simulink model "stellaris_lp_overrun"  (R2017a)
settings: Solver=ode3  StartTime=0.0  StopTime=10.0  FixedStep=1/30e3  RelTol=1e-3
libraries: stellaris_lp_lib x3, simulink x3
settings Model: ExtModeTrigDuration=2  Creator=peselnikmg  LastModifiedBy=Nilim
settings DataIOCC: LimitDataPoints=on  SaveFormat=Array  SignalLoggingSaveFormat=ModelDataLogs
settings OptimizationCC: PassReuseOutputArgsAs=Individual arguments  ExpressionDepthLimit=2147483647  MaxStackSize=64
settings DebuggingCC: ParameterTunabilityLossMsg=error  StateNameClashWarn=warning  SFUnexpectedBacktrackingDiag=warning  SFNoUnconditionalDefaultTransitionDiag=warning  SFExecutionAtInitializationDiag=none
settings HardwareCC: ProdBitPerPointer=32  ProdBitPerSizeT=32  ProdBitPerPtrDiffT=32  ProdLargestAtomicInteger=Long  ProdLargestAtomicFloat=Double  ProdWordSize=32  ProdHWDeviceType=ARM Compatible->ARM Cortex
settings ModelReferenceCC: PropagateSignalLabelsOutOfModel=off
settings SFSimCC: MATLABDynamicMemAlloc=off
settings RTWCC: SystemTargetFile=ert.tlc  HardwareBoard=Tiva TM4C123G Launchpad  TLCOptions=-aInlineSetEventsForThisBaseRateFcn=TLC_FALSE -aSuppressMultiTaskScheduler=TLC_FALSE -aRateBasedStepFcn=1  TemplateMakefile=ert_default_tmf  Description=Embedded Coder  GenerateReport=on  RTWVerbose=off  Toolchain=Texas Instruments Code Composer Studio (Tiva)  IncludeHyperlinkInReport=on  LaunchReport=on  GenerateTraceInfo=on  GenerateTraceReport=on  GenerateTraceReportSl=on  GenerateTraceReportSf=on  GenerateTraceReportEml=on
settings CodeAppCC: ForceParamTrailComments=on  IgnoreCustomStorageClasses=off  OperatorAnnotations=on  SimulinkDataObjDesc=on  SFDataObjDesc=on  MATLABFcnDesc=on  CustomSymbolStrType=$N$R$M  InsertBlockDesc=on  MATLABSourceComments=on  InternalIdentifier=Classic
settings ConfigComp: CovMetricSettings=dw  CovHtmlReporting=on  CovSaveCumulativeToWorkspaceVar=on  CovSaveSingleToWorkspaceVar=on  CovExternalEMLEnable=off

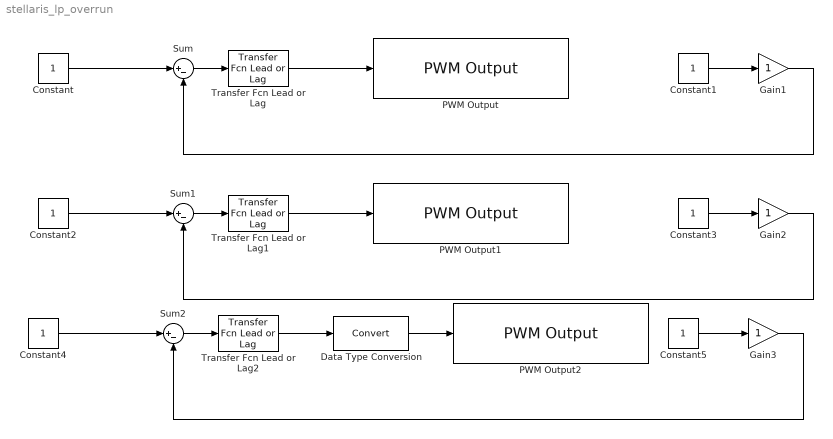
== system stellaris_lp_overrun ==
  Constant : Constant  OutDataTypeStr=single
  Constant1 : Constant  OutDataTypeStr=single  SampleTime=1/30e3
  Constant2 : Constant  OutDataTypeStr=single
  Constant3 : Constant  OutDataTypeStr=single  SampleTime=1/30e3
  Constant4 : Constant  OutDataTypeStr=double
  Constant5 : Constant  OutDataTypeStr=double  SampleTime=1/30e3
  Data Type Conversion : DataTypeConversion
  Gain1 : Gain  OutDataTypeStr=single
  Gain2 : Gain  OutDataTypeStr=single
  Gain3 : Gain  OutDataTypeStr=single
  PWM Output : stellaris_lp_lib/PWM/PWM Output  ch="1    PC4"  invert=off  freq=2e4  sample_time=-1
      settings: SourceProductName=Run on Stellaris LaunchPad
  PWM Output1 : stellaris_lp_lib/PWM/PWM Output  ch="1    PC4"  invert=off  freq=2e4  sample_time=-1
      settings: SourceProductName=Run on Stellaris LaunchPad
  PWM Output2 : stellaris_lp_lib/PWM/PWM Output  ch="1    PC4"  invert=off  freq=2e4  sample_time=-1
      settings: SourceProductName=Run on Stellaris LaunchPad
  Sum : Sum  Inputs=|+-
  Sum1 : Sum  Inputs=|+-
  Sum2 : Sum  Inputs=|+-
  Transfer Fcn Lead or Lag : simulink/Discrete/Transfer Fcn Lead or Lag  PoleZ=0.95  ZeroZ=0.75  ICPrevOutput=0.0  ICPrevInput=0.0  DoSatur=off
      settings: SourceProductName=Simulink  SourceProductBaseCode=SL
  Transfer Fcn Lead or Lag1 : simulink/Discrete/Transfer Fcn Lead or Lag  PoleZ=0.95  ZeroZ=0.75  ICPrevOutput=0.0  ICPrevInput=0.0  DoSatur=off
      settings: SourceProductName=Simulink  SourceProductBaseCode=SL
  Transfer Fcn Lead or Lag2 : simulink/Discrete/Transfer Fcn Lead or Lag  PoleZ=0.95  ZeroZ=0.75  ICPrevOutput=0.0  ICPrevInput=0.0  DoSatur=off
      settings: SourceProductName=Simulink  SourceProductBaseCode=SL
  wires:
  Constant1/1 -> Gain1/1
  Sum/1 -> Transfer Fcn Lead or Lag/1
  Gain1/1 -> Sum/2
  Constant/1 -> Sum/1
  Transfer Fcn Lead or Lag/1 -> PWM Output/1
  Constant3/1 -> Gain2/1
  Sum1/1 -> Transfer Fcn Lead or Lag1/1
  Gain2/1 -> Sum1/2
  Constant2/1 -> Sum1/1
  Transfer Fcn Lead or Lag1/1 -> PWM Output1/1
  Constant5/1 -> Gain3/1
  Sum2/1 -> Transfer Fcn Lead or Lag2/1
  Gain3/1 -> Sum2/2
  Constant4/1 -> Sum2/1
  Transfer Fcn Lead or Lag2/1 -> Data Type Conversion/1
  Data Type Conversion/1 -> PWM Output2/1
